simulink model "control"  (R2020a)
settings: Solver=FixedStepDiscrete  StartTime=0.0  StopTime=1  FixedStep=0.0005  RelTol=1e-3  EnableMultiTasking=on
undefined symbols (not defined in the file): acc_calmax1, acc_calmax2, acc_calmin1, acc_calmin2, akemancanshu, bre, bre_calmax, bre_calmin, ecucoder_acal, I_AN01_5K1, I_AN03_5V, I_AN04_5V, kd, ki, kp, leftmax, O_SW06_HS1A, rightmax, T_add, T_del, tiaoshi, zhiling
libraries: ec5744lib x252, canmsglib x92, simulink x5
(part 6 of 9)

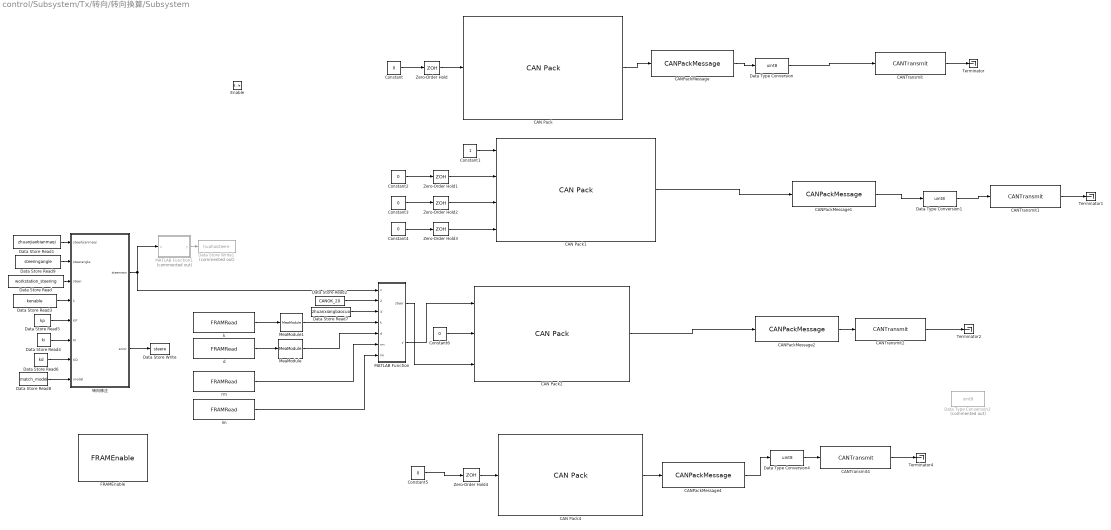
== system control/Subsystem/Tx/转向/转向换算/Subsystem ==
  Enable : EnablePort
  CAN Pack : canmsglib/CAN Pack  CANdbFile=C:\Users\Liu keliang\Desktop\HRT2023\HRT23赛季刘科良\CANdbc\steering.dbc  MsgList=(none)  MsgName=enable123  MsgIDType=Standard (11-bit identifier)  MsgIdentifier=291  MsgLength=1  Remote=off  ApplyMinMax=off  BusOutput=off  SignalInfo={'enable123','0','8','LE','unsigned','Standard','0','1','0','0','255'}
      settings: SourceProductBaseCode=ME,XP,VN  DataFormat=CANdb specified signals
  CAN Pack1 : canmsglib/CAN Pack  CANdbFile=C:\Users\Liu keliang\Desktop\HRT2023\HRT23赛季刘科良\CANdbc\steering.dbc  MsgList=(none)  MsgName=enable0  MsgIDType=Standard (11-bit identifier)  MsgIdentifier=0  MsgLength=8  Remote=off  ApplyMinMax=off  BusOutput=off  SignalInfo={'enable_00','0','16','LE','unsigned','Standard','0','1','0','0','65535';'enable_00_Copy_1','16','16','LE','unsigned','Standard','0','1','0','0','65535';'enable_00_Copy_2','32','16','LE','unsigned','Standard','0','1','0','0','65535';'enable_00_Copy_3','48','16','LE','unsigned','Standard','0','1','0','0','65535'}
      settings: SourceProductBaseCode=ME,XP,VN  DataFormat=CANdb specified signals
  CAN Pack2 : canmsglib/CAN Pack  CANdbFile=C:\Users\Liu keliang\Desktop\HRT2023\HRT23赛季刘科良\CANdbc\steering.dbc  MsgList=(none)  MsgName=enable401  MsgIDType=Standard (11-bit identifier)  MsgIdentifier=1025  MsgLength=6  Remote=off  ApplyMinMax=off  BusOutput=off  SignalInfo={'enable401','0','8','LE','unsigned','Standard','0','1','0','0','255';'enable401_Copy_1','8','8','LE','unsigned','Standard','0','1','0','0','255';'enable401_Copy_2','16','32','LE','signed','Standard','0','1','0','-2147483648','2147483647'}
      settings: SourceProductBaseCode=ME,XP,VN  DataFormat=CANdb specified signals
  CAN Pack4 : canmsglib/CAN Pack  CANdbFile=C:\Users\Liu keliang\Desktop\HRT2023\HRT23赛季刘科良\CANdbc\steering.dbc  MsgList=(none)  MsgName=enable80  MsgIDType=Standard (11-bit identifier)  MsgIdentifier=128  MsgLength=1  Remote=off  ApplyMinMax=off  BusOutput=off  SignalInfo={'dingshi','0','8','LE','unsigned','Standard','0','1','0','0','255'}
      settings: SourceProductBaseCode=ME,XP,VN  DataFormat=CANdb specified signals
  CANPackMessage : ec5744lib/RapidECU_U4B/04CANCommunication/CANPackMessage  datalength=1  sampletime=-1
      settings: SourceProductName=ECUCoder for MPC5744
  CANPackMessage1 : ec5744lib/RapidECU_U4B/04CANCommunication/CANPackMessage  datalength=8  sampletime=-1
      settings: SourceProductName=ECUCoder for MPC5744
  CANPackMessage2 : ec5744lib/RapidECU_U4B/04CANCommunication/CANPackMessage  datalength=6  sampletime=-1
      settings: SourceProductName=ECUCoder for MPC5744
  CANPackMessage4 : ec5744lib/RapidECU_U4B/04CANCommunication/CANPackMessage  datalength=1  sampletime=-1
      settings: SourceProductName=ECUCoder for MPC5744
  CANTransmit : ec5744lib/RapidECU_U4B/04CANCommunication/CANTransmit  canmodule=2  canbuffer=15  canmessageid=hex2dec('123')  canmessagetype=Standard(11-bit ID)  datalength=1  sampletime=-1
      settings: SourceProductName=ECUCoder for MPC5744
  CANTransmit1 : ec5744lib/RapidECU_U4B/04CANCommunication/CANTransmit  canmodule=2  canbuffer=56  canmessageid=hex2dec('00')  canmessagetype=Standard(11-bit ID)  datalength=8  sampletime=-1
      settings: SourceProductName=ECUCoder for MPC5744
  CANTransmit2 : ec5744lib/RapidECU_U4B/04CANCommunication/CANTransmit  canmodule=2  canbuffer=57  canmessageid=hex2dec('401')  canmessagetype=Standard(11-bit ID)  datalength=6  sampletime=-1
      settings: SourceProductName=ECUCoder for MPC5744
  CANTransmit4 : ec5744lib/RapidECU_U4B/04CANCommunication/CANTransmit  canmodule=2  canbuffer=58  canmessageid=hex2dec('80')  canmessagetype=Standard(11-bit ID)  datalength=1  sampletime=-1
      settings: SourceProductName=ECUCoder for MPC5744
  Constant : Constant  Value=0  SampleTime=-1
  Constant1 : Constant  SampleTime=-1
  Constant{2..4,6} (4 alike) : Constant  Value=0
  Constant5 : Constant  Value=0  SampleTime=-1
  Data Store Read : DataStoreRead  DataStoreName=workstation_steering
  Data Store Read1 : DataStoreRead  DataStoreName=zhuanjiaobianmaqi
  Data Store Read2 : DataStoreRead  DataStoreName=CANOK_20
  Data Store Read3 : DataStoreRead  DataStoreName=kenable
  Data Store Read4 : DataStoreRead  DataStoreName=ki
  Data Store Read5 : DataStoreRead  DataStoreName=kp
  Data Store Read6 : DataStoreRead  DataStoreName=kd
  Data Store Read7 : DataStoreRead  DataStoreName=zhuanxiangbaocuo
  Data Store Read8 : DataStoreRead  DataStoreName=match_model
  Data Store Read9 : DataStoreRead  DataStoreName=steeringangle
  Data Store Write : DataStoreWrite  DataStoreName=steere
  Data Store Write1 : DataStoreWrite  Commented=on  DataStoreName=huahaisteere
  Data Type Conversion : DataTypeConversion  OutDataTypeStr=uint8
  Data Type Conversion1 : DataTypeConversion  OutDataTypeStr=uint8
  Data Type Conversion2 : DataTypeConversion  Commented=on  OutDataTypeStr=uint8
  Data Type Conversion4 : DataTypeConversion  OutDataTypeStr=uint8
  FRAMEnable : ec5744lib/RapidECU_U4B/12EEModule/FRAMEnable  framenable=on
      settings: SourceProductName=ECUCoder for MPC5744
  MATLAB Function : MATLAB Function  TreatAsAtomicUnit=on
  MATLAB Function1 : MATLAB Function  Commented=on  TreatAsAtomicUnit=on
  MeaModule : ec5744lib/RapidECU_U4B/07Calibration/MeaModule  signal=d
      settings: SourceProductName=ECUCoder for MPC5744
  MeaModule1 : ec5744lib/RapidECU_U4B/07Calibration/MeaModule  signal=k
      settings: SourceProductName=ECUCoder for MPC5744
  Terminator{,1..2,4} (4 alike) : Terminator
  Zero-Order Hold{,1..4} (5 alike) : ZeroOrderHold  SampleTime=-1
  d : ec5744lib/RapidECU_U4B/12EEModule/FRAMRead  buffer=1  sampletime=-1
      settings: SourceProductName=ECUCoder for MPC5744
  k : ec5744lib/RapidECU_U4B/12EEModule/FRAMRead  buffer=0  sampletime=-1
      settings: SourceProductName=ECUCoder for MPC5744
  lm : ec5744lib/RapidECU_U4B/12EEModule/FRAMRead  buffer=11  sampletime=-1
      settings: SourceProductName=ECUCoder for MPC5744
  rm : ec5744lib/RapidECU_U4B/12EEModule/FRAMRead  buffer=10  sampletime=-1
      settings: SourceProductName=ECUCoder for MPC5744
  转向修正 : MATLAB Function  TreatAsAtomicUnit=on
  wires:
  CANTransmit/1 -> Terminator/1
  Zero-Order Hold2/1 -> CAN Pack1/3
  MATLAB Function/2(y) -> CAN Pack2/1
  CAN Pack1/1 -> CANPackMessage1/1
  CANTransmit2/1 -> Terminator2/1
  CANPackMessage4/1 -> Data Type Conversion4/1
  CAN Pack2/1 -> CANPackMessage2/1
  CANTransmit1/1 -> Terminator1/1
  Constant/1 -> Zero-Order Hold/1
  Data Type Conversion1/1 -> CANTransmit1/1
  Constant6/1 -> CAN Pack2/2
  CANTransmit4/1 -> Terminator4/1
  Data Type Conversion/1 -> CANTransmit/1
  Zero-Order Hold/1 -> CAN Pack/1
  CANPackMessage/1 -> Data Type Conversion/1
  Data Type Conversion4/1 -> CANTransmit4/1
  Constant4/1 -> Zero-Order Hold3/1
  CAN Pack/1 -> CANPackMessage/1
  CANPackMessage1/1 -> Data Type Conversion1/1
  Constant5/1 -> Zero-Order Hold4/1
  CAN Pack4/1 -> CANPackMessage4/1
  Constant3/1 -> Zero-Order Hold2/1
  Constant2/1 -> Zero-Order Hold1/1
  Constant1/1 -> CAN Pack1/1
  Zero-Order Hold4/1 -> CAN Pack4/1
  Zero-Order Hold1/1 -> CAN Pack1/2
  CANPackMessage2/1 -> CANTransmit2/1
  Zero-Order Hold3/1 -> CAN Pack1/4
  MATLAB Function/1(steer) -> CAN Pack2/3
  Data Store Read/1 -> 转向修正/3(steer)
  Data Store Read1/1 -> 转向修正/1(steerbianmaqi)
  转向修正/1(steernew) -> MATLAB Function/1(x), MATLAB Function1/1(u)
  转向修正/2(error) -> Data Store Write/1
  Data Store Read2/1 -> MATLAB Function/2(canok)
  Data Store Read5/1 -> 转向修正/5(KP)
  Data Store Read4/1 -> 转向修正/6(KI)
  Data Store Read3/1 -> 转向修正/4(k)
  Data Store Read6/1 -> 转向修正/7(KD)
  MATLAB Function1/1(y) -> Data Store Write1/1
  Data Store Read7/1 -> MATLAB Function/3(baocuo)
  Data Store Read8/1 -> 转向修正/8(model)
  Data Store Read9/1 -> 转向修正/2(steerangle)
  rm/1 -> MATLAB Function/6(rm)
  lm/1 -> MATLAB Function/7(lm)
  d/1 -> MeaModule/1
  MeaModule/1 -> MATLAB Function/5(d)
  k/1 -> MeaModule1/1
  MeaModule1/1 -> MATLAB Function/4(k)

== system control/Subsystem/Tx/转向/转向换算/Subsystem1 ==
  y1 : Inport
  y2 : Inport  Port=2
  Enable : EnablePort
  CAN Pack5 : canmsglib/CAN Pack  CANdbFile=C:\Users\Liu keliang\Desktop\HRT2023\HRT23赛季刘科良\CANdbc\zhuanxiangresetting.dbc  MsgList=(none)  MsgName=reseting  MsgIDType=Standard (11-bit identifier)  MsgIdentifier=1537  MsgLength=8  Remote=off  ApplyMinMax=off  BusOutput=off  SignalInfo={'reseting1','0','32','LE','unsigned','Standard','0','1','0','-Inf','Inf';'reseting2','32','32','LE','unsigned','Standard','0','1','0','-Inf','Inf'}
      settings: SourceProductBaseCode=ME,XP,VN  DataFormat=CANdb specified signals
  CANPackMessage3 : ec5744lib/RapidECU_U4B/04CANCommunication/CANPackMessage  datalength=8  sampletime=-1
      settings: SourceProductName=ECUCoder for MPC5744
  CANTransmit3 : ec5744lib/RapidECU_U4B/04CANCommunication/CANTransmit  canmodule=2  canbuffer=60  canmessageid=hex2dec('601')  canmessagetype=Standard(11-bit ID)  datalength=8  sampletime=-1
      settings: SourceProductName=ECUCoder for MPC5744
  Data Type Conversion3 : DataTypeConversion  OutDataTypeStr=uint8
  Terminator3 : Terminator
  wires:
  CAN Pack5/1 -> CANPackMessage3/1
  y1/1 -> CAN Pack5/1
  CANTransmit3/1 -> Terminator3/1
  Data Type Conversion3/1 -> CANTransmit3/1
  CANPackMessage3/1 -> Data Type Conversion3/1
  y2/1 -> CAN Pack5/2

== system control/Subsystem/run/analog_input/无人意图转译/无人 ==
  Data Store Write : DataStoreWrite  DataStoreName=escmax
  Max : MinMax  Function=max  Inputs=4
  Subsystem1 : Subsystem
  右前油压 : DataStoreWrite  DataStoreName=oral_pressure_rightfront
  右后油压 : DataStoreWrite  DataStoreName=oral_pressure_rightbehind
  左前油压 : DataStoreWrite  DataStoreName=oral_pressure_leftfront
  左后油压 : DataStoreWrite  DataStoreName=oral_pressure_leftbehind
  期望加速度 : DataStoreWrite  Commented=on  DataStoreName=acc_expired
  期望纵向加速度 : Outport
  wires:
  Subsystem1/1(期望纵向加速度) -> 期望纵向加速度/1, 期望加速度/1
  Subsystem1/2(输出左前制动力) -> Max/1, 左前油压/1
  Subsystem1/4(输出左后制动力) -> Max/3, 左后油压/1
  Subsystem1/3(输出右前制动力) -> Max/2, 右前油压/1
  Subsystem1/5(输出右后制动力) -> Max/4, 右后油压/1
  Max/1 -> Data Store Write/1

== system control/Subsystem/run/analog_input/有人/Subsystem ==
  AnalogInput : ec5744lib/RapidECU_U4B/01BasicInput/AnalogInput  channel=52:I_AN03_5V  sampletime=-1
      settings: SourceProductName=ECUCoder for MPC5744
  AnalogInput1 : ec5744lib/RapidECU_U4B/01BasicInput/AnalogInput  channel=53:I_AN04_5V  sampletime=-1
      settings: SourceProductName=ECUCoder for MPC5744
  AnalogInput2 : ec5744lib/RapidECU_U4B/01BasicInput/AnalogInput  channel=34:I_AN01_5K1  sampletime=-1
      settings: SourceProductName=ECUCoder for MPC5744
  Data Store Write1 : DataStoreWrite  DataStoreName=acc_calibration
  Data Store Write2 : DataStoreWrite  DataStoreName=bre_calibration
  Data Type Conversion : DataTypeConversion  OutDataTypeStr=double
  ECCalVar1 : Constant  InitFcn=ecucoder_acal;  Value=acc_calmax1  OutDataTypeStr=double  SampleTime=-1
  ECCalVar2 : Constant  InitFcn=ecucoder_acal;  Value=acc_calmin1  OutDataTypeStr=double  SampleTime=-1
  ECCalVar3 : Constant  InitFcn=ecucoder_acal;  Value=acc_calmax2  OutDataTypeStr=double  SampleTime=-1
  ECCalVar4 : Constant  InitFcn=ecucoder_acal;  Value=acc_calmin2  OutDataTypeStr=double  SampleTime=-1
  ECCalVar5 : Constant  InitFcn=ecucoder_acal;  Value=bre_calmax  OutDataTypeStr=double  SampleTime=-1
  ECCalVar6 : Constant  InitFcn=ecucoder_acal;  Value=bre_calmin  OutDataTypeStr=double  SampleTime=-1
  ECCalVar7 : Constant  InitFcn=ecucoder_acal;  Value=bre  OutDataTypeStr=double  SampleTime=-1
  FRAMEnable : ec5744lib/RapidECU_U4B/12EEModule/FRAMEnable  Commented=on  framenable=off
      settings: SourceProductName=ECUCoder for MPC5744
  MATLAB Function : MATLAB Function  TreatAsAtomicUnit=on
  MATLAB Function1 : MATLAB Function  TreatAsAtomicUnit=on
  MATLAB Function2 : MATLAB Function  TreatAsAtomicUnit=on
  MeaModule1 : ec5744lib/RapidECU_U4B/07Calibration/MeaModule  signal=acc_ori_line1
      settings: SourceProductName=ECUCoder for MPC5744
  MeaModule2 : ec5744lib/RapidECU_U4B/07Calibration/MeaModule  signal=acc_ori_line2
      settings: SourceProductName=ECUCoder for MPC5744
  MeaModule3 : ec5744lib/RapidECU_U4B/07Calibration/MeaModule  signal=guiyi
      settings: SourceProductName=ECUCoder for MPC5744
  MeaModule5 : ec5744lib/RapidECU_U4B/07Calibration/MeaModule  signal=bre_ori_sig
      settings: SourceProductName=ECUCoder for MPC5744
  MeaModule6 : ec5744lib/RapidECU_U4B/07Calibration/MeaModule  signal=acc_result2
      settings: SourceProductName=ECUCoder for MPC5744
  MeaModule8 : ec5744lib/RapidECU_U4B/07Calibration/MeaModule  signal=acc_result1
      settings: SourceProductName=ECUCoder for MPC5744
  MeaModule9 : ec5744lib/RapidECU_U4B/07Calibration/MeaModule  signal=bre_result
      settings: SourceProductName=ECUCoder for MPC5744
  Subsystem : Subsystem  Commented=on
  Subsystem1 : Subsystem  Commented=on
  无人制动标志位 : DataStoreRead  DataStoreName=wurenzhidongdeng
  踏板冲突 : MATLAB Function  TreatAsAtomicUnit=on
  acc : Outport
  bre : Outport  Port=2
  wires:
  AnalogInput/1 -> MeaModule1/1
  MeaModule8/1 -> 踏板冲突/1(acc_fin_sig1)
  AnalogInput2/1 -> MeaModule5/1
  MeaModule5/1 -> MATLAB Function1/1(u)
  AnalogInput1/1 -> MeaModule2/1
  MeaModule1/1 -> MATLAB Function/1(u)
  MeaModule2/1 -> MATLAB Function2/1(u)
  MeaModule9/1 -> Data Store Write2/1, bre/1, 踏板冲突/3(bre_ori_sig)
  ECCalVar3/1 -> MATLAB Function2/3(max)
  MATLAB Function2/1(y) -> MeaModule6/1
  ECCalVar1/1 -> MATLAB Function/3(max)
  ECCalVar4/1 -> MATLAB Function2/2(min)
  MATLAB Function/1(y) -> MeaModule8/1
  ECCalVar2/1 -> MATLAB Function/2(min)
  Subsystem1/1(y) -> Subsystem/Enable
  MeaModule6/1 -> Data Type Conversion/1
  Data Type Conversion/1 -> 踏板冲突/2(acc_fin_sig2)
  ECCalVar6/1 -> MATLAB Function1/2(min)
  ECCalVar5/1 -> MATLAB Function1/3(max)
  踏板冲突/1(y) -> Data Store Write1/1, MeaModule3/1
  MeaModule3/1 -> acc/1
  ECCalVar7/1 -> 踏板冲突/4(bre)
  无人制动标志位/1 -> MeaModule9/1

== system control/Subsystem/run/analog_input/有人/Subsystem1 ==
  note: 标定
  acc_signal : Inport
  Constant : Constant  Value=0
  Data Store Read : DataStoreRead  DataStoreName=V_Kalman
  Data Type Conversion : DataTypeConversion  OutMin=[0]  OutMax=[1]  OutDataTypeStr=double
  Divide1 : Product  Inputs=**  OutDataTypeStr=uint16
  ECCalVar : Constant  InitFcn=ecucoder_acal;  Value=T_add  OutDataTypeStr=Inherit: Inherit via back propagation  SampleTime=-1
  ECCalVar1 : Constant  InitFcn=ecucoder_acal;  Value=T_del  OutDataTypeStr=Inherit: Inherit via back propagation  SampleTime=-1
  ECCalVar2 : Constant  InitFcn=ecucoder_acal;  Value=zhiling  OutDataTypeStr=Inherit: Inherit via back propagation  SampleTime=-1
  MATLAB Function : MATLAB Function  TreatAsAtomicUnit=on
  MATLAB Function1 : MATLAB Function  TreatAsAtomicUnit=on
  Saturation3 : Saturate  UpperLimit=2100  LowerLimit=0
  Saturation4 : Saturate  UpperLimit=1  LowerLimit=0
  Sum : Sum  Inputs=|++-
  Sum1 : Sum  Inputs=+--
  TP : Outport
  wires:
  Data Type Conversion/1 -> Saturation4/1
  acc_signal/1 -> Data Type Conversion/1
  Saturation4/1 -> Divide1/2
  Sum/1 -> Divide1/1
  ECCalVar1/1 -> Sum/3
  ECCalVar/1 -> Sum/1
  Saturation3/1 -> Sum/2
  Data Store Read/1 -> MATLAB Function/1(v)
  MATLAB Function/1(T) -> Saturation3/1
  Divide1/1 -> Sum1/1
  Constant/1 -> Sum1/2
  Sum1/1 -> MATLAB Function1/1(T)
  MATLAB Function1/1(TP) -> TP/1
  ECCalVar2/1 -> Sum1/3

== system control/Subsystem/run/ctrl/Subsystem1/control_strategy ==
  TP : Inport
  Data Store Read1 : DataStoreRead  DataStoreName=workstation_steering
  Data Store Read2 : DataStoreRead  DataStoreName=slipyouhou
  Data Store Read4 : DataStoreRead  DataStoreName=workstation_steering
  Data Store Read5 : DataStoreRead  DataStoreName=slipzuohou
  Data Store Read6 : DataStoreRead  DataStoreName=slipyuoqian
  Data Store Read7 : DataStoreRead  DataStoreName=slipzuoqian
  E,H : MATLAB Function  Commented=on  TreatAsAtomicUnit=on
  MATLAB Function : MATLAB Function  Commented=on  TreatAsAtomicUnit=on
  MATLAB Function1 : MATLAB Function  TreatAsAtomicUnit=on
  MATLAB Function2 : MATLAB Function  Commented=on  TreatAsAtomicUnit=on
  MATLAB Function3 : MATLAB Function  TreatAsAtomicUnit=on
  MPC : MATLAB Function  Commented=on  TreatAsAtomicUnit=on
  Subsystem : Subsystem  Commented=on
  Switch{,1..3} (4 alike) : Switch  Criteria=u2 > Threshold
  差速 : Subsystem
  滑模控制 : MATLAB Function  TreatAsAtomicUnit=on
  限滑 : Subsystem
  youhou : Outport
  youqian : Outport  Port=2
  zuohou : Outport  Port=3
  zuoqian : Outport  Port=4
  wires:
  TP/1 -> 差速/1(u), 限滑/1(In1)
  Data Store Read4/1 -> MATLAB Function1/1(angle)
  MATLAB Function1/1(y) -> Switch2/2, Switch3/2, Switch1/2, Switch/2
  限滑/1(youhou) -> Switch/3
  限滑/2(youqian) -> Switch1/3
  限滑/3(zuohou) -> Switch2/3
  限滑/4(zuoqian) -> Switch3/3
  MATLAB Function2/1(A) -> E,H/1(A)
  MATLAB Function2/2(B) -> E,H/2(B)
  MATLAB Function2/3(Q) -> E,H/3(Q)
  MATLAB Function2/4(R) -> E,H/4(R)
  MATLAB Function2/5(F) -> E,H/5(F)
  MATLAB Function2/6(N) -> E,H/6(N)
  差速/1(youhou) -> Switch/1
  差速/2(youqian) -> Switch1/1
  差速/3(zuohou) -> Switch2/1
  差速/4(zuoqian) -> Switch3/1
  Data Store Read1/1 -> MATLAB Function3/1(angle)
  MATLAB Function3/1(y) -> 差速/Enable
  Data Store Read7/1 -> 滑模控制/1(slip_ratio_fl)
  Switch/1 -> 滑模控制/8(driver_torque_cmd_rr)
  Data Store Read2/1 -> 滑模控制/4(slip_ratio_rr)
  Data Store Read6/1 -> 滑模控制/2(slip_ratio_fr)
  Switch3/1 -> 滑模控制/5(driver_torque_cmd_fl)
  Data Store Read5/1 -> 滑模控制/3(slip_ratio_rl)
  Switch1/1 -> 滑模控制/6(driver_torque_cmd_fr)
  Switch2/1 -> 滑模控制/7(driver_torque_cmd_rl)
  滑模控制/4(torque_cmd_rr) -> youhou/1
  滑模控制/2(torque_cmd_fr) -> youqian/1
  滑模控制/3(torque_cmd_rl) -> zuohou/1
  滑模控制/1(torque_cmd_fl) -> zuoqian/1

== system control/Subsystem/Rx/工作站/Subsystem1/Subsystem1/Subsystem ==
  ID : Inport
  msg : Inport  Port=2
  CAN Unpack : canmsglib/CAN Unpack  CANdbFile=C:\Users\Liu keliang\Desktop\HRT2023\HRT23赛季刘科良\CANdbc\INSWORKSTATION.dbc  MsgList=(none)  MsgName=ins  MsgIDType=Standard (11-bit identifier)  MsgIdentifier=33  MsgLength=8  SignalInfo={'Vx','32','16','LE','unsigned','Standard','0','1','0','0','65535';'Vy','48','16','LE','unsigned','Standard','0','1','0','0','65535';'ax','0','8','LE','signed','Standard','0','1','0','-128','127';'ay','8','16','LE','signed','Standard','0','1','0','-32768','32767';'az','24','8','LE','signed','Standard','0','1','0','-128','127'}  IDPort=off  TimestampPort=off  ErrorPort=off  RemotePort=off  LengthPort=off  StatusPort=off  ApplyMinMax=off
      settings: SourceProductBaseCode=ME,XP,VN  DataFormat=CANdb specified signals
  CANUnPackMessage : ec5744lib/RapidECU_U4B/04CANCommunication/CANUnPackMessage  datalength=8  canmessagetype=Standard(11-bit ID)  sampletime=-1
      settings: SourceProductName=ECUCoder for MPC5744
  Data Store Write1 : DataStoreWrite  DataStoreName=ACC_X
  Data Store Write2 : DataStoreWrite  DataStoreName=ACC_Y
  Data Store Write3 : DataStoreWrite  DataStoreName=ACC_Z
  Data Store Write4 : DataStoreWrite  DataStoreName=V_Y
  Data Store Write5 : DataStoreWrite  DataStoreName=V_X
  wires:
  msg/1 -> CANUnPackMessage/2
  CANUnPackMessage/1 -> CAN Unpack/1
  ID/1 -> CANUnPackMessage/1
  CAN Unpack/2 -> Data Store Write4/1
  CAN Unpack/1 -> Data Store Write5/1
  CAN Unpack/3 -> Data Store Write1/1
  CAN Unpack/5 -> Data Store Write3/1
  CAN Unpack/4 -> Data Store Write2/1

== system control/Subsystem/Rx/工作站/Subsystem3/Subsystem/Subsystem ==
  Data Store Read : DataStoreRead  DataStoreName=CANOK_20
  Delay : Delay  DelayLength=1
  Delay1 : Delay
  Delay10 : Delay  DelayLength=11
  Delay11 : Delay  DelayLength=12
  Delay12 : Delay  DelayLength=13
  Delay13 : Delay  DelayLength=14
  Delay14 : Delay  DelayLength=15
  Delay15 : Delay  DelayLength=16
  Delay16 : Delay  DelayLength=17
  Delay17 : Delay  DelayLength=25
  Delay18 : Delay  DelayLength=18
  Delay19 : Delay  DelayLength=19
  Delay2 : Delay  DelayLength=3
  Delay20 : Delay  DelayLength=20
  Delay21 : Delay  DelayLength=21
  Delay22 : Delay  DelayLength=22
  Delay23 : Delay  DelayLength=26
  Delay24 : Delay  DelayLength=24
  Delay25 : Delay  DelayLength=27
  Delay3 : Delay  DelayLength=4
  Delay4 : Delay  DelayLength=5
  Delay5 : Delay  DelayLength=6
  Delay6 : Delay  DelayLength=7
  Delay7 : Delay  DelayLength=8
  Delay8 : Delay  DelayLength=9
  Delay9 : Delay  DelayLength=10
  OR : Logic  Operator=OR  Inputs=27  IconShape=distinctive  AllPortsSameDT=off  OutDataTypeStr=boolean
  Out1 : Outport
  wires:
  Delay2/1 -> OR/2
  Delay/1 -> OR/4
  Data Store Read/1 -> Delay23/1, Delay25/1, Delay17/1, Delay24/1, Delay22/1, Delay21/1, Delay20/1, Delay19/1, Delay18/1, Delay16/1, Delay15/1, Delay14/1, Delay13/1, Delay12/1, Delay11/1, Delay10/1, Delay8/1, Delay6/1, Delay5/1, Delay7/1, Delay9/1, OR/5, Delay3/1, Delay2/1, Delay1/1, Delay/1, Delay4/1
  Delay5/1 -> OR/7
  Delay1/1 -> OR/3
  Delay9/1 -> OR/11
  Delay7/1 -> OR/9
  Delay3/1 -> OR/1
  Delay8/1 -> OR/8
  Delay6/1 -> OR/6
  Delay4/1 -> OR/10
  OR/1 -> Out1/1
  Delay10/1 -> OR/12
  Delay11/1 -> OR/13
  Delay12/1 -> OR/14
  Delay13/1 -> OR/15
  Delay14/1 -> OR/16
  Delay15/1 -> OR/17
  Delay16/1 -> OR/18
  Delay18/1 -> OR/19
  Delay19/1 -> OR/20
  Delay20/1 -> OR/21
  Delay21/1 -> OR/22
  Delay22/1 -> OR/23
  Delay24/1 -> OR/24
  Delay17/1 -> OR/25
  Delay23/1 -> OR/27
  Delay25/1 -> OR/26

== system control/Subsystem/Tx/TX控制器/扭矩/TEST/Subsystem ==
  Enable : EnablePort
  CAN Pack1 : canmsglib/CAN Pack  CANdbFile=C:\Users\Liu keliang\Desktop\HRT2023\HRT23赛季刘科良\CANdbc\TEST.dbc  MsgList=(none)  MsgName=TEST  MsgIDType=Standard (11-bit identifier)  MsgIdentifier=153  MsgLength=5  Remote=off  ApplyMinMax=off  BusOutput=off  SignalInfo={'M','16','8','LE','signed','Standard','0','1','0','-Inf','Inf';'X2D','32','8','LE','signed','Standard','0','1','0','-Inf','Inf';'a','0','8','LE','signed','Standard','0','1','0','-Inf','Inf';'deltv','8','8','LE','signed','Standard','0','1','0','-Inf','Inf';'niuju','24','8','LE','signed','Standard','0','1','0','-Inf','Inf'}
      settings: SourceProductBaseCode=ME,XP,VN  DataFormat=CANdb specified signals
  CANPackMessage1 : ec5744lib/RapidECU_U4B/04CANCommunication/CANPackMessage  datalength=5  sampletime=-1
      settings: SourceProductName=ECUCoder for MPC5744
  CANTransmit : ec5744lib/RapidECU_U4B/04CANCommunication/CANTransmit  canmodule=0  canbuffer=63  canmessageid=hex2dec('99')  canmessagetype=Standard(11-bit ID)  datalength=5  sampletime=-1
      settings: SourceProductName=ECUCoder for MPC5744
  Data Store Read : DataStoreRead  DataStoreName=a
  Data Store Read1 : DataStoreRead  DataStoreName=ve
  Data Store Read2 : DataStoreRead  DataStoreName=M
  Data Store Read3 : DataStoreRead  DataStoreName=acc
  Data Store Read4 : DataStoreRead  DataStoreName=dianji_velcoity_zuoqian
  Data Type Conversion1 : DataTypeConversion  OutDataTypeStr=uint8
  Terminator : Terminator
  wires:
  Data Store Read4/1 -> CAN Pack1/1
  CANTransmit/1 -> Terminator/1
  Data Store Read3/1 -> CAN Pack1/3
  CANPackMessage1/1 -> Data Type Conversion1/1
  Data Store Read2/1 -> CAN Pack1/5
  Data Type Conversion1/1 -> CANTransmit/1
  Data Store Read1/1 -> CAN Pack1/4
  Data Store Read/1 -> CAN Pack1/2
  CAN Pack1/1 -> CANPackMessage1/1

== system control/Subsystem/Tx/TX控制器/速度1/184左前/能量回收功率限制 ==
  note: U
  note: Iq
  Constant1 : Constant  Value=2
  Constant24 : Constant  Value=1000
  Data Store Read1 : DataStoreRead  DataStoreName=er_T_lf
  Data Store Read2 : DataStoreRead  DataStoreName=match_model
  Data Store Read25 : DataStoreRead  DataStoreName=er_v_lf
  Data Store Read3 : DataStoreRead  DataStoreName=oral_pressure_leftfront
  Data Store Read8 : DataStoreRead  DataStoreName=workstation_status
  Divide : Product  Inputs=*/
  Divide1 : Product  Inputs=***/
  Divide2 : Product  Inputs=**
  Gain : Gain  Gain=100
  MATLAB Function : MATLAB Function  TreatAsAtomicUnit=on
  MATLAB Function1 : MATLAB Function  TreatAsAtomicUnit=on
  Sqrt : Sqrt  SaturateOnIntegerOverflow=on
  功率限制P : Constant  Value=500
  扭矩常量Kr  N/A : Constant  Value=0.26
  油压传感器 : DataStoreRead  DataStoreName=ebszhidongyouya
  电压常数Ke V/kU/min : Constant  Value=18.8
  T : Outport
  wires:
  Data Store Read25/1 -> Divide1/1
  电压常数Ke V/kU/min/1 -> Divide1/2
  Constant24/1 -> Divide1/4
  Sqrt/1 -> Divide1/3
  Constant1/1 -> Sqrt/1
  油压传感器/1 -> MATLAB Function/1(youya)
  功率限制P/1 -> Divide/1
  Divide1/1 -> Divide/2
  Divide/1 -> MATLAB Function1/3(L_Iq), Divide2/1
  扭矩常量Kr  N/A/1 -> Divide2/2
  MATLAB Function/1(T) -> MATLAB Function1/1(er_T)
  Data Store Read1/1 -> MATLAB Function1/2(Iq)
  Divide2/1 -> Gain/1
  Gain/1 -> MATLAB Function1/4(L_er_T)
  MATLAB Function1/1(T) -> T/1
  Data Store Read2/1 -> MATLAB Function/2(model)
  Data Store Read8/1 -> MATLAB Function/3(status)
  Data Store Read3/1 -> MATLAB Function/4(wurenyouya)

== system control/Subsystem/Tx/TX控制器/速度1/185右前/能量回收功率限制 ==
  note: U
  note: Iq
  Constant1 : Constant  Value=2
  Constant24 : Constant  Value=1000
  Data Store Read1 : DataStoreRead  DataStoreName=er_T_rf
  Data Store Read2 : DataStoreRead  DataStoreName=match_model
  Data Store Read25 : DataStoreRead  DataStoreName=er_v_rf
  Data Store Read3 : DataStoreRead  DataStoreName=oral_pressure_rightfront
  Data Store Read8 : DataStoreRead  DataStoreName=workstation_status
  Divide : Product  Inputs=*/
  Divide1 : Product  Inputs=***/
  Divide2 : Product  Inputs=**
  Gain : Gain  Gain=100
  MATLAB Function : MATLAB Function  TreatAsAtomicUnit=on
  MATLAB Function1 : MATLAB Function  TreatAsAtomicUnit=on
  Sqrt : Sqrt  SaturateOnIntegerOverflow=on
  功率限制P : Constant  Value=500
  扭矩常量Kr  N/A : Constant  Value=0.26
  油压传感器 : DataStoreRead  DataStoreName=ebszhidongyouya
  电压常数Ke V/kU/min : Constant  Value=18.8
  T : Outport
  wires:
  Data Store Read25/1 -> Divide1/1
  电压常数Ke V/kU/min/1 -> Divide1/2
  Constant24/1 -> Divide1/4
  Sqrt/1 -> Divide1/3
  Constant1/1 -> Sqrt/1
  功率限制P/1 -> Divide/1
  Divide1/1 -> Divide/2
  Divide/1 -> MATLAB Function1/3(L_Iq), Divide2/1
  扭矩常量Kr  N/A/1 -> Divide2/2
  MATLAB Function/1(T) -> MATLAB Function1/1(er_T)
  Data Store Read1/1 -> MATLAB Function1/2(Iq)
  Divide2/1 -> Gain/1
  Gain/1 -> MATLAB Function1/4(L_er_T)
  MATLAB Function1/1(T) -> T/1
  油压传感器/1 -> MATLAB Function/1(youya)
  Data Store Read3/1 -> MATLAB Function/4(wurenyouya)
  Data Store Read8/1 -> MATLAB Function/3(status)
  Data Store Read2/1 -> MATLAB Function/2(model)

== system control/Subsystem/Tx/TX控制器/速度1/188右后/能量回收功率限制 ==
  note: U
  note: Iq
  Constant1 : Constant  Value=2
  Constant24 : Constant  Value=1000
  Data Store Read1 : DataStoreRead  DataStoreName=er_T_rb
  Data Store Read2 : DataStoreRead  DataStoreName=match_model
  Data Store Read25 : DataStoreRead  DataStoreName=er_v_rb
  Data Store Read3 : DataStoreRead  DataStoreName=oral_pressure_rightbehind
  Data Store Read8 : DataStoreRead  DataStoreName=workstation_status
  Divide : Product  Inputs=*/
  Divide1 : Product  Inputs=***/
  Divide2 : Product  Inputs=**
  Gain : Gain  Gain=100
  MATLAB Function : MATLAB Function  TreatAsAtomicUnit=on
  MATLAB Function1 : MATLAB Function  TreatAsAtomicUnit=on
  Sqrt : Sqrt  SaturateOnIntegerOverflow=on
  功率限制P : Constant  Value=500
  扭矩常量Kr  N/A : Constant  Value=0.26
  油压传感器 : DataStoreRead  DataStoreName=ebszhidongyouya
  电压常数Ke V/kU/min : Constant  Value=18.8
  T : Outport
  wires:
  Data Store Read25/1 -> Divide1/1
  电压常数Ke V/kU/min/1 -> Divide1/2
  Constant24/1 -> Divide1/4
  Sqrt/1 -> Divide1/3
  Constant1/1 -> Sqrt/1
  功率限制P/1 -> Divide/1
  Divide1/1 -> Divide/2
  Divide/1 -> MATLAB Function1/3(L_Iq), Divide2/1
  扭矩常量Kr  N/A/1 -> Divide2/2
  MATLAB Function/1(T) -> MATLAB Function1/1(er_T)
  Data Store Read1/1 -> MATLAB Function1/2(Iq)
  Divide2/1 -> Gain/1
  Gain/1 -> MATLAB Function1/4(L_er_T)
  MATLAB Function1/1(T) -> T/1
  油压传感器/1 -> MATLAB Function/1(youya)
  Data Store Read3/1 -> MATLAB Function/4(wurenyouya)
  Data Store Read8/1 -> MATLAB Function/3(status)
  Data Store Read2/1 -> MATLAB Function/2(model)

== system control/Subsystem/Tx/TX控制器/速度1/189左后/能量回收功率限制 ==
  note: U
  note: Iq
  Constant1 : Constant  Value=2
  Constant24 : Constant  Value=1000
  Data Store Read1 : DataStoreRead  DataStoreName=er_T_lb
  Data Store Read2 : DataStoreRead  DataStoreName=match_model
  Data Store Read25 : DataStoreRead  DataStoreName=er_v_lb
  Data Store Read3 : DataStoreRead  DataStoreName=oral_pressure_leftbehind
  Data Store Read8 : DataStoreRead  DataStoreName=workstation_status
  Divide : Product  Inputs=*/
  Divide1 : Product  Inputs=***/
  Divide2 : Product  Inputs=**
  Gain : Gain  Gain=100
  MATLAB Function : MATLAB Function  TreatAsAtomicUnit=on
  MATLAB Function1 : MATLAB Function  TreatAsAtomicUnit=on
  Sqrt : Sqrt  SaturateOnIntegerOverflow=on
  功率限制P : Constant  Value=500
  扭矩常量Kr  N/A : Constant  Value=0.26
  油压传感器 : DataStoreRead  DataStoreName=ebszhidongyouya
  电压常数Ke V/kU/min : Constant  Value=18.8
  T : Outport
  wires:
  Data Store Read25/1 -> Divide1/1
  电压常数Ke V/kU/min/1 -> Divide1/2
  Constant24/1 -> Divide1/4
  Sqrt/1 -> Divide1/3
  Constant1/1 -> Sqrt/1
  功率限制P/1 -> Divide/1
  Divide1/1 -> Divide/2
  Divide/1 -> MATLAB Function1/3(L_Iq), Divide2/1
  扭矩常量Kr  N/A/1 -> Divide2/2
  MATLAB Function/1(T) -> MATLAB Function1/1(er_T)
  Data Store Read1/1 -> MATLAB Function1/2(Iq)
  Divide2/1 -> Gain/1
  Gain/1 -> MATLAB Function1/4(L_er_T)
  MATLAB Function1/1(T) -> T/1
  油压传感器/1 -> MATLAB Function/1(youya)
  Data Store Read3/1 -> MATLAB Function/4(wurenyouya)
  Data Store Read8/1 -> MATLAB Function/3(status)
  Data Store Read2/1 -> MATLAB Function/2(model)

== system control/Subsystem/Tx/Toworkstation/转向/Subsystem/Subsystem ==
  Enable : EnablePort
  CAN Pack : canmsglib/CAN Pack  CANdbFile=C:\Users\Liu keliang\Desktop\HRT2023\HRT23赛季刘科良\CANdbc\steering.dbc  MsgList=(none)  MsgName=enable123  MsgIDType=Standard (11-bit identifier)  MsgIdentifier=291  MsgLength=1  Remote=off  ApplyMinMax=off  BusOutput=off  SignalInfo={'enable123','0','8','LE','unsigned','Standard','0','1','0','0','255'}
      settings: SourceProductBaseCode=ME,XP,VN  DataFormat=CANdb specified signals
  CAN Pack1 : canmsglib/CAN Pack  CANdbFile=C:\Users\Liu keliang\Desktop\HRT2023\HRT23赛季刘科良\CANdbc\steering.dbc  MsgList=(none)  MsgName=enable0  MsgIDType=Standard (11-bit identifier)  MsgIdentifier=0  MsgLength=8  Remote=off  ApplyMinMax=off  BusOutput=off  SignalInfo={'enable_00','0','16','LE','unsigned','Standard','0','1','0','0','65535';'enable_00_Copy_1','16','16','LE','unsigned','Standard','0','1','0','0','65535';'enable_00_Copy_2','32','16','LE','unsigned','Standard','0','1','0','0','65535';'enable_00_Copy_3','48','16','LE','unsigned','Standard','0','1','0','0','65535'}
      settings: SourceProductBaseCode=ME,XP,VN  DataFormat=CANdb specified signals
  CAN Pack2 : canmsglib/CAN Pack  CANdbFile=C:\Users\Liu keliang\Desktop\HRT2023\HRT23赛季刘科良\CANdbc\steering.dbc  MsgList=(none)  MsgName=enable401  MsgIDType=Standard (11-bit identifier)  MsgIdentifier=1025  MsgLength=6  Remote=off  ApplyMinMax=off  BusOutput=off  SignalInfo={'enable401','0','8','LE','unsigned','Standard','0','1','0','0','255';'enable401_Copy_1','8','8','LE','unsigned','Standard','0','1','0','0','255';'enable401_Copy_2','16','32','LE','signed','Standard','0','1','0','-2147483648','2147483647'}
      settings: SourceProductBaseCode=ME,XP,VN  DataFormat=CANdb specified signals
  CAN Pack4 : canmsglib/CAN Pack  CANdbFile=C:\Users\Liu keliang\Desktop\HRT2023\HRT23赛季刘科良\CANdbc\steering.dbc  MsgList=(none)  MsgName=enable80  MsgIDType=Standard (11-bit identifier)  MsgIdentifier=128  MsgLength=1  Remote=off  ApplyMinMax=off  BusOutput=off  SignalInfo={'dingshi','0','8','LE','unsigned','Standard','0','1','0','0','255'}
      settings: SourceProductBaseCode=ME,XP,VN  DataFormat=CANdb specified signals
  CANPackMessage : ec5744lib/RapidECU_U4B/04CANCommunication/CANPackMessage  datalength=1  sampletime=-1
      settings: SourceProductName=ECUCoder for MPC5744
  CANPackMessage1 : ec5744lib/RapidECU_U4B/04CANCommunication/CANPackMessage  datalength=8  sampletime=-1
      settings: SourceProductName=ECUCoder for MPC5744
  CANPackMessage2 : ec5744lib/RapidECU_U4B/04CANCommunication/CANPackMessage  datalength=6  sampletime=-1
      settings: SourceProductName=ECUCoder for MPC5744
  CANPackMessage4 : ec5744lib/RapidECU_U4B/04CANCommunication/CANPackMessage  datalength=1  sampletime=-1
      settings: SourceProductName=ECUCoder for MPC5744
  CANTransmit : ec5744lib/RapidECU_U4B/04CANCommunication/CANTransmit  canmodule=2  canbuffer=15  canmessageid=hex2dec('123')  canmessagetype=Standard(11-bit ID)  datalength=1  sampletime=-1
      settings: SourceProductName=ECUCoder for MPC5744
  CANTransmit1 : ec5744lib/RapidECU_U4B/04CANCommunication/CANTransmit  canmodule=2  canbuffer=56  canmessageid=hex2dec('00')  canmessagetype=Standard(11-bit ID)  datalength=8  sampletime=-1
      settings: SourceProductName=ECUCoder for MPC5744
  CANTransmit2 : ec5744lib/RapidECU_U4B/04CANCommunication/CANTransmit  canmodule=2  canbuffer=57  canmessageid=hex2dec('401')  canmessagetype=Standard(11-bit ID)  datalength=6  sampletime=-1
      settings: SourceProductName=ECUCoder for MPC5744
  CANTransmit4 : ec5744lib/RapidECU_U4B/04CANCommunication/CANTransmit  canmodule=2  canbuffer=58  canmessageid=hex2dec('80')  canmessagetype=Standard(11-bit ID)  datalength=1  sampletime=-1
      settings: SourceProductName=ECUCoder for MPC5744
  Constant : Constant  Value=0  SampleTime=-1
  Constant1 : Constant  SampleTime=-1
  Constant{2..4,6} (4 alike) : Constant  Value=0
  Constant5 : Constant  Value=0  SampleTime=-1
  Data Type Conversion{,1..2,4} (4 alike) : DataTypeConversion  OutDataTypeStr=uint8
  MATLAB Function : MATLAB Function  TreatAsAtomicUnit=on
  Saturation : Saturate  UpperLimit=758000  LowerLimit=605000
  Terminator{,1..2,4} (4 alike) : Terminator
  Zero-Order Hold{,1..4} (5 alike) : ZeroOrderHold  SampleTime=-1
  wires:
  CANTransmit/1 -> Terminator/1
  Zero-Order Hold2/1 -> CAN Pack1/3
  MATLAB Function/2(y) -> CAN Pack2/1
  CAN Pack1/1 -> CANPackMessage1/1
  CANTransmit2/1 -> Terminator2/1
  CANPackMessage4/1 -> Data Type Conversion4/1
  CAN Pack2/1 -> CANPackMessage2/1
  CANTransmit1/1 -> Terminator1/1
  Constant/1 -> Zero-Order Hold/1
  Data Type Conversion1/1 -> CANTransmit1/1
  Constant6/1 -> CAN Pack2/2
  CANTransmit4/1 -> Terminator4/1
  Data Type Conversion/1 -> CANTransmit/1
  Zero-Order Hold/1 -> CAN Pack/1
  CANPackMessage2/1 -> Data Type Conversion2/1
  CANPackMessage/1 -> Data Type Conversion/1
  Data Type Conversion4/1 -> CANTransmit4/1
  Constant4/1 -> Zero-Order Hold3/1
  CAN Pack/1 -> CANPackMessage/1
  CANPackMessage1/1 -> Data Type Conversion1/1
  Constant5/1 -> Zero-Order Hold4/1
  CAN Pack4/1 -> CANPackMessage4/1
  Constant3/1 -> Zero-Order Hold2/1
  Constant2/1 -> Zero-Order Hold1/1
  Constant1/1 -> CAN Pack1/1
  Zero-Order Hold4/1 -> CAN Pack4/1
  MATLAB Function/1(steer) -> Saturation/1
  Zero-Order Hold1/1 -> CAN Pack1/2
  Data Type Conversion2/1 -> CANTransmit2/1
  Zero-Order Hold3/1 -> CAN Pack1/4
  Saturation/1 -> CAN Pack2/3

== system control/Subsystem/Tx/Toworkstation/转向/Subsystem/Subsystem1 ==
  y1 : Inport
  y2 : Inport  Port=2
  Enable : EnablePort
  CAN Pack5 : canmsglib/CAN Pack  CANdbFile=C:\Users\Liu keliang\Desktop\HRT2023\HRT23赛季刘科良\CANdbc\zhuanxiangresetting.dbc  MsgList=(none)  MsgName=reseting  MsgIDType=Standard (11-bit identifier)  MsgIdentifier=1537  MsgLength=8  Remote=off  ApplyMinMax=off  BusOutput=off  SignalInfo={'reseting1','0','32','LE','unsigned','Standard','0','1','0','-Inf','Inf';'reseting2','32','32','LE','unsigned','Standard','0','1','0','-Inf','Inf'}
      settings: SourceProductBaseCode=ME,XP,VN  DataFormat=CANdb specified signals
  CANPackMessage3 : ec5744lib/RapidECU_U4B/04CANCommunication/CANPackMessage  datalength=8  sampletime=-1
      settings: SourceProductName=ECUCoder for MPC5744
  CANTransmit3 : ec5744lib/RapidECU_U4B/04CANCommunication/CANTransmit  canmodule=2  canbuffer=61  canmessageid=hex2dec('601')  canmessagetype=Standard(11-bit ID)  datalength=8  sampletime=-1
      settings: SourceProductName=ECUCoder for MPC5744
  Data Type Conversion3 : DataTypeConversion  OutDataTypeStr=uint8
  Terminator3 : Terminator
  wires:
  CAN Pack5/1 -> CANPackMessage3/1
  y1/1 -> CAN Pack5/1
  CANTransmit3/1 -> Terminator3/1
  Data Type Conversion3/1 -> CANTransmit3/1
  CANPackMessage3/1 -> Data Type Conversion3/1
  y2/1 -> CAN Pack5/2

== system control/Subsystem/run/analog_input/无人意图转译/无人/Subsystem1 ==
  note: 希望在反馈delta，但是不知道为啥生成代码，所以先置0
  note: 灵感忘了，怎么用忘了，暂且保留，也可以当观测器
  note: 输出期望加速度,进控制策略
  note: 进esc控制策略
  note: u(3)=e（暂时不用）
      | u(4)=K1
      | u(5)=K2
      | u(6)=delta（暂时不用）
      | u(7)=x1
      | u(8)=x2
      | u(9)=x1d
      | u(10)=dotx1d
      | u(11)=ddotx1d
  note: delta
  note: e
  note: 此处判断加减速
  note: 实车测试用下面六个口
  note: u(1)=dotx1d
      | u(2)=e
      | u(3)=K1
      | u(4)=delta
      | u(5)=k2
  Add : Sum
  Add1 : Sum
  Constant : Constant  Value=0
  Data Store Read : DataStoreRead  DataStoreName=V_workstation
  Data Store Read1 : DataStoreRead  DataStoreName=ve
  Data Store Read15 : DataStoreRead  Commented=on  DataStoreName=velcolity_min
  Data Store Read19 : DataStoreRead  DataStoreName=oilyouqian
  Data Store Read20 : DataStoreRead  DataStoreName=oilyouhou
  Data Store Read21 : DataStoreRead  DataStoreName=oilzuohou
  Data Store Read22 : DataStoreRead  DataStoreName=oilzuoqian
  Data Store Read4 : DataStoreRead  DataStoreName=ACC_X
  Data Store Read9 : DataStoreRead  DataStoreName=V_Kalman
  Data Store Write : DataStoreWrite  Commented=on  DataStoreName=a
  Data Store Write1 : DataStoreWrite  DataStoreName=ve
  Delay : Delay
  Delay1 : Delay  DelayLength=3
  Delay2 : Delay  DelayLength=4
  Desired : Subsystem
  "Input " : Scope  Commented=on
  K1 : Constant  Value=0.5
  K2 : Constant  Value=0.3
  MATLAB Function : MATLAB Function  TreatAsAtomicUnit=on
  MATLAB Function3 : MATLAB Function  TreatAsAtomicUnit=on
  Mux : Mux  Commented=on  Inputs=2
  Mux2 : Mux  Inputs=5
  Mux3 : Mux  Commented=on  Inputs=11
  Saturation{,1..3} (4 alike) : Saturate  UpperLimit=4500  LowerLimit=0
  Saturation{4..7} (4 alike) : Saturate  UpperLimit=2100  LowerLimit=0
  Subsystem : Subsystem
  Sum1 : Sum  Inputs=|+-
  X2d : Fcn  Expr=u(1)+u(3)*u(2)+u(4)*u(5)
  dotx2 : Sum  Commented=on  Inputs=|++
  id : MATLAB Function  TreatAsAtomicUnit=on
  tiaoshi : Constant  InitFcn=ecucoder_acal;  Value=tiaoshi  OutDataTypeStr=double  SampleTime=-1
  u : Fcn  Commented=on  Expr=(1+u(4)*u(5)+u(5))*u(9)-(1+u(4)*u(5))*u(7)-(u(4)+u(5)-1)*u(8)+u(4)*u(10)+u(11)
  x1 : Integrator  Commented=on
  x1d x1 : Scope  Commented=on
  x2 : Integrator  Commented=on  UpperSaturationLimit=10  ZeroCross=off
  x2d,x2 : Scope  Commented=on  NumInputPorts=3
  计算四轮各自制动力 : Subsystem
  计算油压 : MATLAB Function  TreatAsAtomicUnit=on
  期望纵向加速度 : Outport
  输出左前制动力 : Outport  Port=2
  输出右前制动力 : Outport  Port=3
  输出左后制动力 : Outport  Port=4
  输出右后制动力 : Outport  Port=5
  tag scope: A=global
  wires:
  K2/1 -> Mux2/5, Mux3/5
  计算油压/1(p1) -> Saturation/1
  MATLAB Function/1(y) -> id/1(u), Data Store Write1/1, Mux2/2, [A]
  Desired/4(输入整车加速度测量值x2) -> Sum1/2
  x2/1 -> dotx2/1, x2d,x2/3, x1/1, Mux3/8
  Sum1/1 -> Mux3/6
  计算油压/2(p2) -> Saturation1/1
  MATLAB Function3/2(y2) -> Subsystem/1(期望加速度（负值）)
  计算四轮各自制动力/1(输出左前的制动力) -> Saturation4/1, 计算油压/1(y1)
  Mux/1 -> x1d x1/1
  u/1 -> dotx2/2, "Input "/1
  计算油压/3(p3) -> Saturation2/1
  计算四轮各自制动力/3(输出左后轮的制动力3) -> Saturation6/1, 计算油压/3(y3)
  计算油压/4(p4) -> Saturation3/1
  计算四轮各自制动力/4(输出右后轮的制动力1) -> Saturation7/1, 计算油压/4(y4)
  Subsystem/1(总制动力) -> 计算四轮各自制动力/1(u)
  K1/1 -> Mux2/3, Mux3/4
  dotx2/1 -> x2/1
  Mux2/1 -> X2d/1
  Mux3/1 -> u/1
  x1/1 -> Mux/2, Mux3/7
  Data Store Read9/1 -> Desired/3(输入整车车速测量值1)
  Data Store Read4/1 -> Desired/2(输入整车加速度测量值1)
  X2d/1 -> x2d,x2/2, Sum1/1, Add/1
  Constant/1 -> Mux2/4
  MATLAB Function3/1(y1) -> Data Store Write/1, 期望纵向加速度/1
  Desired/3(x1d输入) -> Subsystem/2(x1d输入), MATLAB Function/1(u)
  Desired/2(dotx1d输入) -> Mux2/1
  tiaoshi/1 -> Add1/1
  Data Store Read/1 -> Add1/2
  Add1/1 -> Desired/1(此处输入感知的期望整车纵向速度), MATLAB Function3/3(vd)
  Desired/5(输入整车车速测量值x1) -> Subsystem/3(输入整车车速测量值x1), MATLAB Function3/2(v), MATLAB Function/2(u2)
  Add/1 -> Delay1/1, Delay2/1, Delay/1, MATLAB Function3/1(u)
  Delay/1 -> MATLAB Function3/4(ade)
  Delay1/1 -> MATLAB Function3/5(adede)
  Delay2/1 -> MATLAB Function3/6(adedede)
  id/1(output) -> Add/2
  Data Store Read20/1 -> 计算油压/8(youhou)
  Data Store Read21/1 -> 计算油压/7(zuohou)
  Data Store Read22/1 -> 计算油压/5(zuoqian)
  Data Store Read19/1 -> 计算油压/6(youqian)
  Data Store Read1/1 -> 计算油压/9(error)
  计算四轮各自制动力/2(输出右前的制动力2) -> 计算油压/2(y2), Saturation5/1
  Saturation4/1 -> 输出左前制动力/1
  Saturation5/1 -> 输出右前制动力/1
  Saturation6/1 -> 输出左后制动力/1
  Saturation7/1 -> 输出右后制动力/1

== system control/Subsystem/run/analog_input/有人/Subsystem/Subsystem ==
  Enable : EnablePort
  Data Type Conversion{,1,4..7} (6 alike) : DataTypeConversion  OutDataTypeStr=single
  ECCalVar1 : Constant  InitFcn=ecucoder_acal;  Value=acc_calmax1  OutDataTypeStr=double  SampleTime=-1
  ECCalVar2 : Constant  InitFcn=ecucoder_acal;  Value=acc_calmin1  OutDataTypeStr=double  SampleTime=-1
  ECCalVar3 : Constant  InitFcn=ecucoder_acal;  Value=acc_calmax2  OutDataTypeStr=double  SampleTime=-1
  ECCalVar4 : Constant  InitFcn=ecucoder_acal;  Value=acc_calmin2  OutDataTypeStr=double  SampleTime=-1
  ECCalVar5 : Constant  InitFcn=ecucoder_acal;  Value=bre_calmax  OutDataTypeStr=double  SampleTime=-1
  ECCalVar6 : Constant  InitFcn=ecucoder_acal;  Value=bre_calmin  OutDataTypeStr=double  SampleTime=-1
  FRAMEnable : ec5744lib/RapidECU_U4B/12EEModule/FRAMEnable  framenable=off
      settings: SourceProductName=ECUCoder for MPC5744
  FRAMWrite1 : ec5744lib/RapidECU_U4B/12EEModule/FRAMWrite  buffer=6  sampletime=-1
      settings: SourceProductName=ECUCoder for MPC5744
  FRAMWrite2 : ec5744lib/RapidECU_U4B/12EEModule/FRAMWrite  buffer=4  sampletime=-1
      settings: SourceProductName=ECUCoder for MPC5744
  FRAMWrite3 : ec5744lib/RapidECU_U4B/12EEModule/FRAMWrite  buffer=5  sampletime=-1
      settings: SourceProductName=ECUCoder for MPC5744
  FRAMWrite4 : ec5744lib/RapidECU_U4B/12EEModule/FRAMWrite  buffer=7  sampletime=-1
      settings: SourceProductName=ECUCoder for MPC5744
  FRAMWrite5 : ec5744lib/RapidECU_U4B/12EEModule/FRAMWrite  buffer=8  sampletime=-1
      settings: SourceProductName=ECUCoder for MPC5744
  FRAMWrite6 : ec5744lib/RapidECU_U4B/12EEModule/FRAMWrite  buffer=9  sampletime=-1
      settings: SourceProductName=ECUCoder for MPC5744
  wires:
  ECCalVar2/1 -> Data Type Conversion/1
  Data Type Conversion/1 -> FRAMWrite5/1
  ECCalVar5/1 -> Data Type Conversion7/1
  Data Type Conversion7/1 -> FRAMWrite3/1
  Data Type Conversion6/1 -> FRAMWrite2/1
  ECCalVar6/1 -> Data Type Conversion6/1
  ECCalVar3/1 -> Data Type Conversion5/1
  Data Type Conversion5/1 -> FRAMWrite4/1
  ECCalVar4/1 -> Data Type Conversion4/1
  Data Type Conversion4/1 -> FRAMWrite1/1
  ECCalVar1/1 -> Data Type Conversion1/1
  Data Type Conversion1/1 -> FRAMWrite6/1

== system control/Subsystem/run/analog_input/有人/Subsystem/Subsystem1 ==
  ECCalVar1 : Constant  InitFcn=ecucoder_acal;  Value=acc_calmax1  OutDataTypeStr=double  SampleTime=-1
  ECCalVar2 : Constant  InitFcn=ecucoder_acal;  Value=acc_calmin1  OutDataTypeStr=double  SampleTime=-1
  ECCalVar3 : Constant  InitFcn=ecucoder_acal;  Value=acc_calmax2  OutDataTypeStr=double  SampleTime=-1
  ECCalVar4 : Constant  InitFcn=ecucoder_acal;  Value=acc_calmin2  OutDataTypeStr=double  SampleTime=-1
  ECCalVar5 : Constant  InitFcn=ecucoder_acal;  Value=bre_calmax  OutDataTypeStr=double  SampleTime=-1
  ECCalVar6 : Constant  InitFcn=ecucoder_acal;  Value=bre_calmin  OutDataTypeStr=double  SampleTime=-1
  MATLAB Function : MATLAB Function  TreatAsAtomicUnit=on
  Max : MinMax  Function=max  Inputs=6
  y : Outport
  wires:
  ECCalVar3/1 -> Max/4
  ECCalVar2/1 -> Max/1
  ECCalVar4/1 -> Max/3
  ECCalVar5/1 -> Max/6
  ECCalVar1/1 -> Max/2
  ECCalVar6/1 -> Max/5
  Max/1 -> MATLAB Function/1(u)
  MATLAB Function/1(y) -> y/1

== system control/Subsystem/run/ctrl/Subsystem1/control_strategy/Subsystem ==
  alpha : Inport
  beta : Inport  Port=2
  -1~1 : Saturate  Commented=on  UpperLimit=1  LowerLimit=-1
  0~5 : Saturate  Commented=on  UpperLimit=5  LowerLimit=0
  Mux : Mux  Commented=on  Inputs=3
  Mux1 : Mux  Commented=on  Inputs=5
  Mux2 : Mux  Commented=on  Inputs=5
  Rules : Subsystem  Commented=on
  Scope alpha : Scope  Commented=on
  Scope beta : Scope  Commented=on
  Scope delta : Scope  Commented=on
  Scope delta sets : Scope  Commented=on
  a1 : Constant  Commented=on  Value=1.2
  a2 : Constant  Commented=on  Value=2.4
  alpha test : simulink/Sources/Ramp  Commented=on  slope=0.1  start=0  InitialOutput=-0.5
  b1 : Constant  Commented=on  Value=-0.5
  b2 : Constant  Commented=on  Value=0
  b3 : Constant  Commented=on  Value=0.5
  beta test : simulink/Sources/Ramp  Commented=on  slope=0.1  start=0  InitialOutput=-1.5
  d1 : Constant  Commented=on  Value=-0.5
  d2 : Constant  Commented=on  Value=0
  d3 : Constant  Commented=on  Value=0.5
  defuzzification : MATLAB Function  Commented=on  TreatAsAtomicUnit=on
  α sets : MATLAB Function  Commented=on  TreatAsAtomicUnit=on
  β sets : MATLAB Function  Commented=on  TreatAsAtomicUnit=on
  delta : Outport  VectorParamsAs1DForOutWhenUnconnected=off
  wires:
  defuzzification/1(delta) -> delta/1, Scope delta/1  "delta"
  Rules/3(do) -> Mux2/3, defuzzification/3(do)
  Rules/5(dpb) -> Mux2/5, defuzzification/5(dpb)
  beta/1 -> -1~1/1
  b3/1 -> β sets/4(b3)
  α sets/1(as) -> Mux/1, Rules/1(as)  "as"
  β sets/3(bo) -> Mux1/3, Rules/6(bo)  "bo"
  d2/1 -> defuzzification/7(d2)
  Rules/4(dps) -> Mux2/4, defuzzification/4(dps)
  β sets/1(bnb) -> Mux1/1, Rules/4(bnb)  "bnb"
  Rules/2(dns) -> Mux2/2, defuzzification/2(dns)
  Mux/1 -> Scope alpha/1
  d1/1 -> defuzzification/6(d1)
  Mux2/1 -> Scope delta sets/1
  β sets/2(bns) -> Mux1/2, Rules/5(bns)  "bns"
  β sets/5(bpb) -> Mux1/5, Rules/8(bpb)  "bpb"
  0~5/1 -> α sets/1(alpha)
  a1/1 -> α sets/2(a1)
  alpha/1 -> 0~5/1
  β sets/4(bps) -> Mux1/4, Rules/7(bps)  "bps"
  Rules/1(dnb) -> Mux2/1, defuzzification/1(dnb)
  Mux1/1 -> Scope beta/1
  -1~1/1 -> β sets/1(beta)
  b2/1 -> β sets/3(b2)
  b1/1 -> β sets/2(b1)
  a2/1 -> α sets/3(a2)
  α sets/2(am) -> Mux/2, Rules/2(am)
  d3/1 -> defuzzification/8(d3)
  α sets/3(ab) -> Mux/3, Rules/3(ab)  "ab"

== system control/Subsystem/run/ctrl/Subsystem1/control_strategy/差速 ==
  u : Inport
  Enable : EnablePort
  MATLAB Function3 : MATLAB Function  TreatAsAtomicUnit=on
  差速 : Subsystem
  youhou : Outport
  youqian : Outport  Port=2
  zuohou : Outport  Port=3
  zuoqian : Outport  Port=4
  wires:
  MATLAB Function3/3(zuohou) -> zuohou/1
  MATLAB Function3/4(zuoqian) -> zuoqian/1
  差速/1(M) -> MATLAB Function3/2(M)
  MATLAB Function3/2(youqian) -> youqian/1
  u/1 -> MATLAB Function3/1(u)
  MATLAB Function3/1(youhou) -> youhou/1

== system control/Subsystem/run/ctrl/Subsystem1/control_strategy/限滑 ==
  In1 : Inport
  MATLAB Function : MATLAB Function  Commented=on  TreatAsAtomicUnit=on
  MPC : Subsystem
  PID限滑 : Subsystem
  Subsystem1 : Subsystem
  youhou : Outport
  youqian : Outport  Port=2
  zuohou : Outport  Port=3
  zuoqian : Outport  Port=4
  wires:
  MPC/2(左后) -> Subsystem1/8(mpc)
  PID限滑/2(throttle_youqian) -> Subsystem1/6(throttle_youqian)
  In1/1 -> PID限滑/1(u), Subsystem1/10(In7), MPC/4(左前in), Subsystem1/1(TP), MPC/1(右后in), Subsystem1/7(u), MPC/2(左后in), Subsystem1/4(In4), MPC/3(右前in)
  MPC/3(右前) -> Subsystem1/5(右前)
  PID限滑/4(throttle_zuoqian) -> Subsystem1/12(throttle_zuoqian)
  PID限滑/3(throttle_zuohou) -> Subsystem1/9(pid)
  MPC/1(右后) -> Subsystem1/2(右后)
  MPC/4(左前) -> Subsystem1/11(左前)
  PID限滑/1(throttle_youhou) -> Subsystem1/3(throttle_youhou)
  Subsystem1/1(youhou) -> youhou/1
  Subsystem1/4(zuoqian) -> zuoqian/1
  Subsystem1/3(zuohou) -> zuohou/1
  Subsystem1/2(youqian) -> youqian/1
